simulink model "q"  (R2018a)
settings: Solver=VariableStepAuto  StartTime=0.0  StopTime=10.0  RelTol=1e-3
settings Model: Creator=master  LastModifiedBy=master

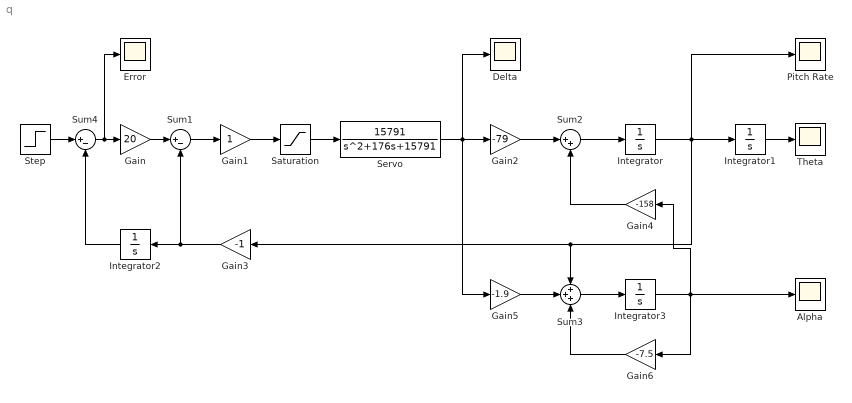
== system q ==
  Alpha : Scope
  Delta : Scope
  Error : Scope
  Gain : Gain  Gain=20
  Gain1 : Gain
  Gain2 : Gain  Gain=-79
  Gain3 : Gain  Gain=-1
  Gain4 : Gain  Gain=-158
  Gain5 : Gain  Gain=-1.9
  Gain6 : Gain  Gain=-7.5
  Integrator{,1..3} (4 alike) : Integrator
  Pitch Rate : Scope
  Saturation : Saturate
  Servo : TransferFcn  Numerator=[15791]  Denominator=[1 176 15791]  ContinuousStateAttributes='Servo'
  Step : Step  SampleTime=0
  Sum1 : Sum  Inputs=|+-
  Sum2 : Sum  Inputs=|++
  Sum3 : Sum  Inputs=+++
  Sum4 : Sum  Inputs=|+-
  Theta : Scope
  wires:
  Sum4/1 -> Gain/1, Error/1
  Gain/1 -> Sum1/1
  Sum1/1 -> Gain1/1
  Gain1/1 -> Saturation/1
  Saturation/1 -> Servo/1
  Servo/1 -> Gain5/1, Delta/1, Gain2/1
  Gain2/1 -> Sum2/1
  Sum2/1 -> Integrator/1
  Integrator/1 -> Sum3/1, Gain3/1, Integrator1/1, Pitch Rate/1
  Integrator1/1 -> Theta/1
  Integrator2/1 -> Sum4/2
  Gain3/1 -> Integrator2/1, Sum1/2
  Gain4/1 -> Sum2/2
  Gain5/1 -> Sum3/2
  Sum3/1 -> Integrator3/1
  Integrator3/1 -> Gain6/1, Alpha/1, Gain4/1
  Gain6/1 -> Sum3/3
  Step/1 -> Sum4/1
